simulink model "PBL3_week3"  (R2020a)
settings: Solver=VariableStepAuto  StartTime=0.0  StopTime=10.0  RelTol=1e-3
model workspace (MAT data in the model file):
  K1 = Simulink.Parameter
  K1.Value = 50
  K1.DataType = 'auto'
  K1.Dimensions = [1 1]
  K12 = Simulink.Parameter
  K12.Value = 40
  K12.DataType = 'auto'
  K12.Dimensions = [1 1]
  M1 = Simulink.Parameter
  M1.Value = 100
  M1.DataType = 'auto'
  M1.Dimensions = [1 1]
  M2 = Simulink.Parameter
  M2.Value = 80
  M2.DataType = 'auto'
  M2.Dimensions = [1 1]
  b = Simulink.Parameter
  b.Value = 50
  b.DataType = 'auto'
  b.Dimensions = [1 1]
settings Model: Creator=hp  LastModifiedBy=hp

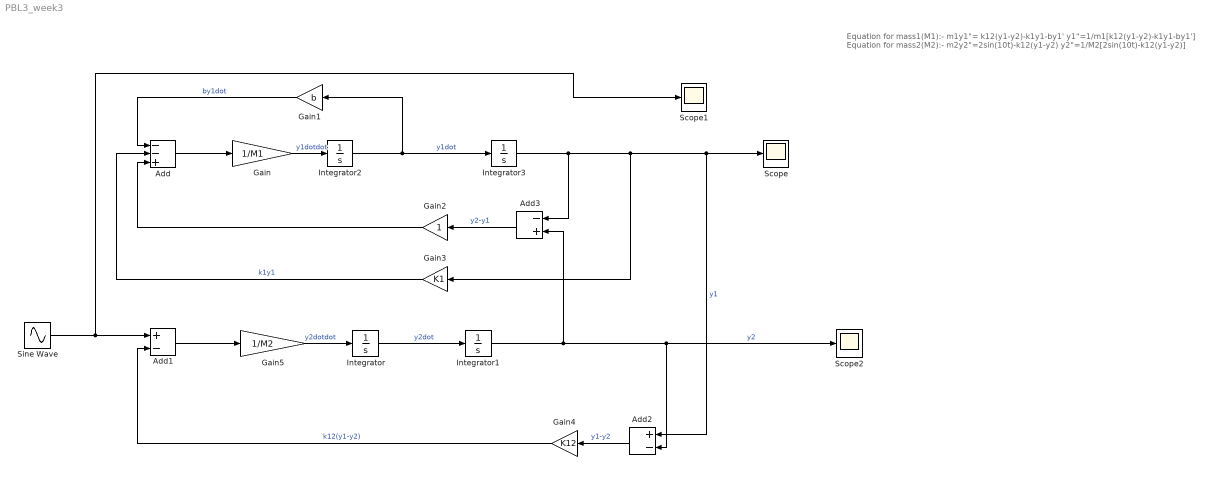
== system PBL3_week3 ==
  note: Equation for mass1(M1):-
      | m1y1"= k12(y1-y2)-k1y1-by1'
      |
      | y1"=1/m1[k12(y1-y2)-k1y1-by1']
      |
      | Equation for mass2(M2):-
      | m2y2"=2sin(10t)-k12(y1-y2)
      |
      | y2"=1/M2[2sin(10t)-k12(y1-y2)]
  Add : Sum  Inputs=--+
  Add1 : Sum  Inputs=+-
  Add2 : Sum  Inputs=+-
  Add3 : Sum  Inputs=-+
  Gain : Gain  Gain=1/M1
  Gain1 : Gain  Gain=b
  Gain2 : Gain
  Gain3 : Gain  Gain=K1
  Gain4 : Gain  Gain=K12
  Gain5 : Gain  Gain=1/M2
  Integrator{,1..3} (4 alike) : Integrator
  Scope : Scope
  Scope1 : Scope
  Scope2 : Scope
  Sine Wave : Sin  SampleTime=0
  wires:
  Add/1 -> Gain/1
  Gain/1 -> Integrator2/1  "y1dotdot"
  Gain4/1 -> Add1/2  "k12(y1-y2)"
  Gain3/1 -> Add/2  "k1y1"
  Add2/1 -> Gain4/1  "y1-y2"
  Gain5/1 -> Integrator/1  "y2dotdot"
  Sine Wave/1 -> Scope1/1, Add1/1
  Gain2/1 -> Add/3
  Integrator3/1 -> Add3/1, Gain3/1, Add2/1, Scope/1  "y1"
  Add3/1 -> Gain2/1  "y2-y1"
  Add1/1 -> Gain5/1
  Integrator/1 -> Integrator1/1  "y2dot"
  Integrator1/1 -> Add2/2, Scope2/1, Add3/2  "y2"
  Integrator2/1 -> Gain1/1, Integrator3/1  "y1dot"
  Gain1/1 -> Add/1  "by1dot"
